simulink model "controller_integral_stateFB"  (R2022b)
settings: Solver=ode4  StartTime=0.0  StopTime=inf  RelTol=1e-3  EnableMultiTasking=on
values from neighbouring files (symbols this model uses):
  KI = Ke(:, 13:end)    [integral_state_feedback.m]
  KP = Ke(:, 1:12)    [integral_state_feedback.m]
  mixer_matrix = [ 1  1  1  1 ... (first row only)    [load_model_parameters.m]
  SampleTime = 0.002    [load_model_parameters.m]
undefined symbols (not defined in the file or in its folder): dev, DiscIntNeverNeededParam, Main, pwm_output0
libraries: px4uORBlib x4, sharedtransform x1, px4lib x1, sharedutil x1
settings Model: ExtModeTrigDuration=10  Creator=paolo  LastModifiedBy=paolo
settings SolverCC: PositivePriorityOrder=on
settings OptimizationCC: EnhancedBackFolding=on  PassReuseOutputArgsAs=Individual arguments  ZeroExternalMemoryAtStartup=off  ZeroInternalMemoryAtStartup=off  MaxStackSize=64  OptimizeBlockOrder=speed  DifferentSizesBufferReuse=on  OptimizationCustomize=off  EfficientTunableParamExpr=on
settings DebuggingCC: ParameterTunabilityLossMsg=error
settings HardwareCC: ProdBitPerPointer=32  ProdBitPerSizeT=32  ProdBitPerPtrDiffT=32  ProdLargestAtomicInteger=Long  ProdLargestAtomicFloat=Double  ProdWordSize=32  ProdLongLongMode=on  ProdHWDeviceType=ARM Compatible->ARM Cortex
settings SFSimCC: MATLABDynamicMemAlloc=off  SimTargetLang=C++
settings RTWCC: Description=Embedded Coder  SystemTargetFile=ert.tlc  HardwareBoard=PX4 Pixracer  TLCOptions="-aInlineSetEventsForThisBaseRateFcn=TLC_FALSE -aSuppressMultiTaskScheduler=TLC_FALSE  -aRateBasedStepFcn=0"  TemplateMakefile=ert_default_tmf  Toolchain=GNU Tools for PX4 Autopilots  TargetLang=C++
settings CodeAppCC: ForceParamTrailComments=on  IgnoreCustomStorageClasses=off  OperatorAnnotations=on  SimulinkDataObjDesc=on  SFDataObjDesc=on  InsertBlockDesc=on
settings ERTTargetCC: ExtModeTransport=3  ExtModeStaticAlloc=on  ExtModeStaticAllocSize=1024  ExtModeMexFile=ext_xcp  ExtModeIntrfLevel=Level2 - Open

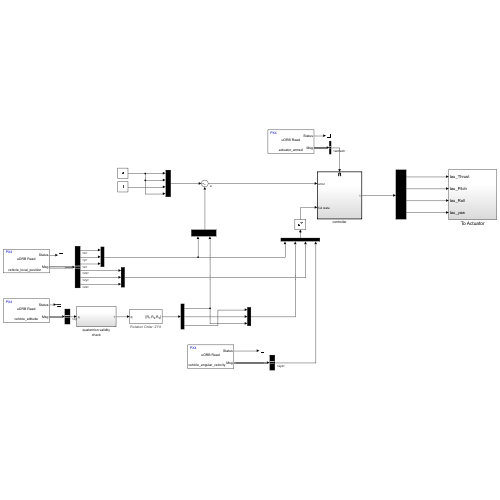
[thumbnail: Simulink's stored preview of the top-level diagram]
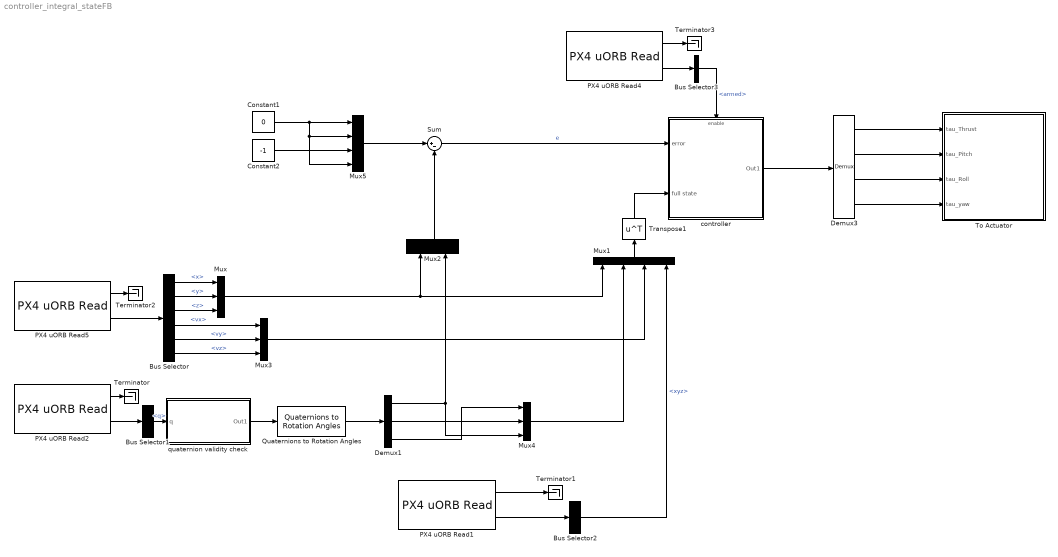
== system controller_integral_stateFB ==
  Bus Selector : BusSelector  OutputSignals=x,y,z,vx,vy,vz
  Bus Selector1 : BusSelector  OutputSignals=q
  Bus Selector2 : BusSelector  OutputSignals=xyz
  Bus Selector3 : BusSelector  OutputSignals=armed
  Constant1 : Constant  Value=0  OutDataTypeStr=single
  Constant2 : Constant  Value=-1  OutDataTypeStr=single  SampleTime=-1
  Demux1 : Demux  Outputs=3
  Demux3 : Demux
  Mux : Mux  Inputs=3
  Mux1 : Mux
  Mux2 : Mux  Inputs=2
  Mux3 : Mux  Inputs=3
  Mux4 : Mux  Inputs=3
  Mux5 : Mux
  PX4 uORB Read1 : px4uORBlib/PX4 uORB Read  uORBTopic=vehicle_angular_velocity  selectInstance=vehicle_angular_velocity  SampleTime=SampleTime  BlockingMode=off  BlockTimeout=1e-3
  PX4 uORB Read2 : px4uORBlib/PX4 uORB Read  uORBTopic=vehicle_attitude  selectInstance=vehicle_attitude  SampleTime=SampleTime  BlockingMode=off  BlockTimeout=1e-3
  PX4 uORB Read4 : px4uORBlib/PX4 uORB Read  uORBTopic=actuator_armed  selectInstance=actuator_armed  SampleTime=SampleTime  BlockingMode=off  BlockTimeout=1e-3
  PX4 uORB Read5 : px4uORBlib/PX4 uORB Read  uORBTopic=vehicle_local_position  selectInstance=vehicle_local_position  SampleTime=SampleTime  BlockingMode=off  BlockTimeout=1e-3
  Quaternions to Rotation Angles : sharedtransform/Quaternions to Rotation Angles  rotationOrder=ZYX  aMode=aMode
  Sum : Sum  Inputs=|+-
  Terminator{,1..3} (4 alike) : Terminator
  To Actuator : Subsystem
  Transpose1 : Math  Operator=transpose
  controller : Subsystem
  quaternion validity check : Subsystem
  wires:
  Demux3/1 -> To Actuator/1(tau_Thrust)
  Demux1/2 -> Mux4/2
  PX4 uORB Read2/1 -> Terminator/1
  Mux5/1 -> Sum/1
  Demux3/3 -> To Actuator/3(tau_Roll)
  Demux3/4 -> To Actuator/4(tau_yaw)
  PX4 uORB Read5/2 -> Bus Selector/1
  Demux1/3 -> Mux4/1
  Demux1/1 -> Mux2/2, Mux4/3
  PX4 uORB Read2/2 -> Bus Selector1/1
  Demux3/2 -> To Actuator/2(tau_Pitch)
  Mux2/1 -> Sum/2
  Bus Selector/1 -> Mux/1  "<x>"
  Bus Selector/2 -> Mux/2  "<y>"
  Bus Selector/3 -> Mux/3  "<z>"
  Bus Selector/5 -> Mux3/2  "<vy>"
  Bus Selector/4 -> Mux3/1  "<vx>"
  Bus Selector/6 -> Mux3/3  "<vz>"
  PX4 uORB Read1/1 -> Terminator1/1
  PX4 uORB Read1/2 -> Bus Selector2/1
  Mux1/1 -> Transpose1/1
  Mux/1 -> Mux2/1, Mux1/1
  Mux3/1 -> Mux1/3
  Mux4/1 -> Mux1/2
  Bus Selector2/1 -> Mux1/4  "<xyz>"
  PX4 uORB Read5/1 -> Terminator2/1
  PX4 uORB Read4/1 -> Terminator3/1
  PX4 uORB Read4/2 -> Bus Selector3/1
  controller/1(Out1) -> Demux3/1
  Bus Selector1/1 -> quaternion validity check/1(q)  "<q>"
  quaternion validity check/1(Out1) -> Quaternions to Rotation Angles/1
  Quaternions to Rotation Angles/1 -> Demux1/1
  Bus Selector3/1 -> controller/Enable  "<armed>"
  Sum/1 -> controller/1(error)  "e"
  Transpose1/1 -> controller/2(full state)
  Constant2/1 -> Mux5/3
  Constant1/1 -> Mux5/4, Mux5/2, Mux5/1

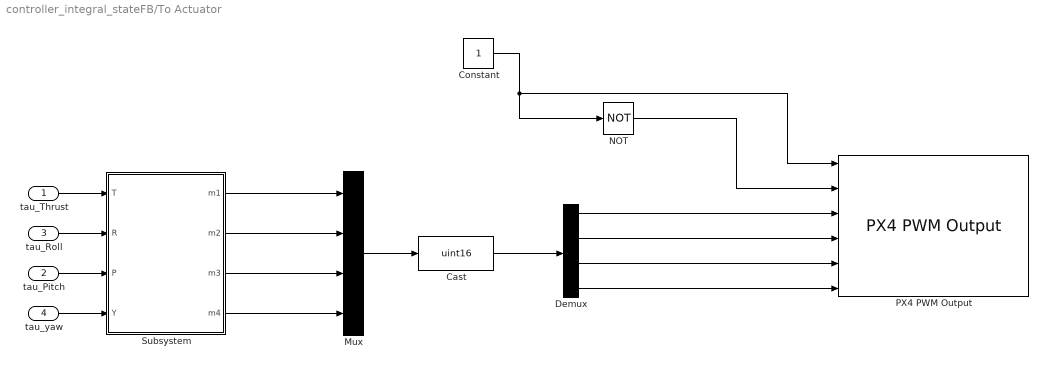
== system controller_integral_stateFB/To Actuator ==
  tau_Thrust : Inport
  tau_Pitch : Inport  Port=2
  tau_Roll : Inport  Port=3
  tau_yaw : Inport  Port=4
  Cast : DataTypeConversion  OutDataTypeStr=uint16  SaturateOnIntegerOverflow=off  RndMeth=Floor
  Constant : Constant  OutDataTypeStr=boolean
  Demux : Demux
  Mux : Mux
  NOT : Logic  Operator=NOT  IconShape=distinctive  AllPortsSameDT=off  OutDataTypeStr=boolean
  PX4 PWM Output : px4lib/PX4 PWM Output  pwmDevice=Main (/dev/pwm_output0)  pwmChannel1_=on  pwmChannel2_=on  pwmChannel3_=on  pwmChannel4_=on  pwmChannel5_=off  pwmChannel6_=off  pwmChannel7_=off  pwmChannel8_=off  forceTerminateFailsafe=off  outputErrorStatus=off
  Subsystem : Subsystem
  wires:
  Mux/1 -> Cast/1
  Subsystem/4(m4) -> Mux/4
  Subsystem/3(m3) -> Mux/3
  Subsystem/1(m1) -> Mux/1
  Subsystem/2(m2) -> Mux/2
  tau_Thrust/1 -> Subsystem/1(T)
  tau_yaw/1 -> Subsystem/4(Y)
  tau_Roll/1 -> Subsystem/2(R)
  tau_Pitch/1 -> Subsystem/3(P)
  NOT/1 -> PX4 PWM Output/2
  Constant/1 -> NOT/1, PX4 PWM Output/1
  Demux/1 -> PX4 PWM Output/3
  Demux/2 -> PX4 PWM Output/4
  Demux/3 -> PX4 PWM Output/5
  Demux/4 -> PX4 PWM Output/6
  Cast/1 -> Demux/1

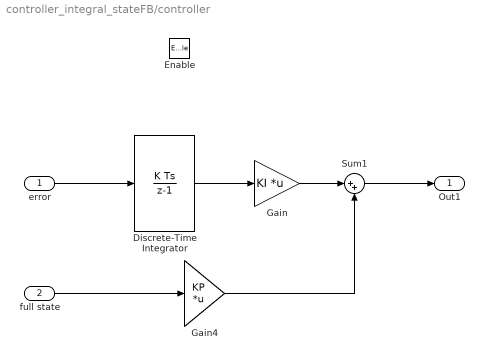
== system controller_integral_stateFB/controller ==
  error : Inport
  full state : Inport  Port=2
  Enable : EnablePort
  Discrete-Time Integrator : DiscreteIntegrator  gainval=1  SampleTime=-1  ICPrevOutput=DiscIntNeverNeededParam  ICPrevScaledInput=DiscIntNeverNeededParam
  Gain : Gain  Gain=KI  Multiplication=Matrix(K*u)
  Gain4 : Gain  Gain=KP  Multiplication=Matrix(K*u)
  Sum1 : Sum  Inputs=|++
  Out1 : Outport
  wires:
  Discrete-Time Integrator/1 -> Gain/1
  Gain4/1 -> Sum1/2
  Gain/1 -> Sum1/1
  Sum1/1 -> Out1/1
  full state/1 -> Gain4/1
  error/1 -> Discrete-Time Integrator/1

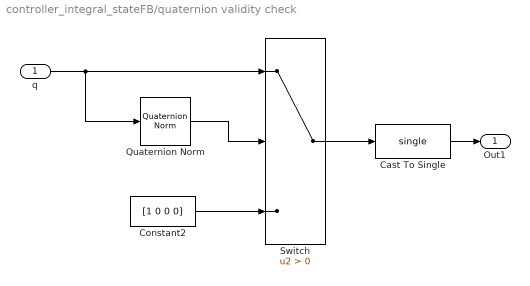
== system controller_integral_stateFB/quaternion validity check ==
  q : Inport
  Cast To Single : DataTypeConversion  OutDataTypeStr=single  SaturateOnIntegerOverflow=off  RndMeth=Floor
  Constant2 : Constant  Value=[1 0 0 0]  SampleTime=-1
  Quaternion Norm : sharedutil/Quaternion Norm  aMode=aMode
  Switch : Switch  Criteria=u2 > Threshold  SaturateOnIntegerOverflow=off  InputSameDT=off
  Out1 : Outport
  wires:
  Constant2/1 -> Switch/3
  Switch/1 -> Cast To Single/1
  Quaternion Norm/1 -> Switch/2
  q/1 -> Quaternion Norm/1, Switch/1
  Cast To Single/1 -> Out1/1

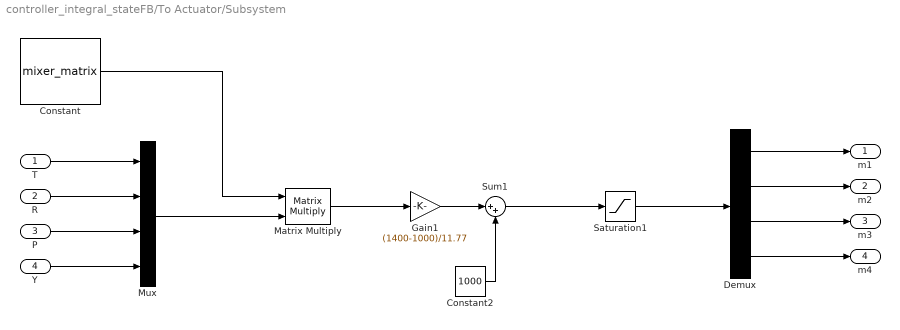
== system controller_integral_stateFB/To Actuator/Subsystem ==
  T : Inport
  R : Inport  Port=2
  P : Inport  Port=3
  Y : Inport  Port=4
  Constant : Constant  Value=mixer_matrix
  Constant2 : Constant  Value=1000
  Demux : Demux
  Gain1 : Gain  Gain=(1400-1000)/11.77
  Matrix Multiply : Product  Multiplication=Matrix(*)
  Mux : Mux
  Saturation1 : Saturate  UpperLimit=2000  LowerLimit=1000
  Sum1 : Sum  Inputs=|++
  m1 : Outport
  m2 : Outport  Port=2
  m3 : Outport  Port=3
  m4 : Outport  Port=4
  wires:
  Saturation1/1 -> Demux/1
  Matrix Multiply/1 -> Gain1/1
  Gain1/1 -> Sum1/1
  Constant2/1 -> Sum1/2
  Sum1/1 -> Saturation1/1
  Demux/4 -> m4/1
  Demux/3 -> m3/1
  Demux/2 -> m2/1
  Demux/1 -> m1/1
  Y/1 -> Mux/4
  R/1 -> Mux/2
  P/1 -> Mux/3
  T/1 -> Mux/1
  Mux/1 -> Matrix Multiply/2
  Constant/1 -> Matrix Multiply/1
